simulink model "NMPC_6DoF_v1"  (R2022b)
settings: Solver=ode45  StartTime=0.0  StopTime=30  FixedStep=0.01  RelTol=1e-3
undefined symbols (not defined in the file): beta, e0_0, e1_0, e2_0, e3_0, eul0, G0, gamma, gc, geometry, Js, Js0, K_lqrq, m_dry, m_fuel, m_full, m_max, mass, omega0, pos0, r_cg, rcgs, ref_eul, Tensors, vel0
libraries: sharedtransform x27, simulink_extras x21, matrix_library x12, sharedutil x2, sharedTrackingLibrary x1, mpclib x1
(part 2 of 2)

== system NMPC_6DoF_v1/6DOF HopperDynamic/Rocket Dynamics 6DOF2/Calculate omega_dot ==
  p q r : Inport
  "I, I_dot" : Inport  Port=2
  Moments : Inport  Port=3
  3x3 Cross Product : sharedutil/3x3 Cross Product  aMode=aMode
  I x w : Subsystem
  I x w1 : Subsystem
  Product2 : Product  Inputs=*/  Multiplication=Matrix(*)  SaturateOnIntegerOverflow=on  OutDataTypeStr=Inherit: Same as first input
  Reshape : Reshape
  Reshape1 : Reshape  OutputDimensionality=Row vector (2-D)
  Selector : Selector  NumberOfDimensions=2  InputPortWidth=2  IndexOptions=Index vector (dialog),Select all  Indices=1:3,-1  OutputSizes=1
  Selector1 : Selector  NumberOfDimensions=2  InputPortWidth=2  IndexOptions=Index vector (dialog),Select all  Indices=4:6,-1  OutputSizes=1
  Selector2 : Selector  NumberOfDimensions=2  InputPortWidth=2  IndexOptions=Index vector (dialog),Select all  Indices=1:3,-1  OutputSizes=1
  Sum2 : Sum  Inputs=+--  SaturateOnIntegerOverflow=on
  pdot qdot rdot : Outport  VectorParamsAs1DForOutWhenUnconnected=off
  wires:
  "I, I_dot"/1 -> Selector1/1, Selector2/1, Selector/1
  Selector/1 -> I x w/2(Inertia)
  I x w/1(I * w) -> 3x3 Cross Product/2
  p q r/1 -> I x w1/2(p q r), 3x3 Cross Product/1, I x w/1(p q r)
  Moments/1 -> Sum2/1
  I x w1/1(Id * w) -> Sum2/2
  3x3 Cross Product/1 -> Sum2/3
  Sum2/1 -> Reshape1/1
  Reshape/1 -> pdot qdot rdot/1
  Selector2/1 -> Product2/2
  Reshape1/1 -> Product2/1
  Product2/1 -> Reshape/1
  Selector1/1 -> I x w1/1(I_dot)

== system NMPC_6DoF_v1/6DOF HopperDynamic/Rocket Dynamics 6DOF2/Determine Force, Mass & Inertia ==
  forces : Inport
  "mass " : Inport  Port=2
  I : Inport  Port=3
  I_dot : Inport  Port=4
  Matrix Concatenation : Concatenate  Mode=Multidimensional array
  "forces " : Outport  PortDimensions=3  VectorParamsAs1DForOutWhenUnconnected=off
  mass : Outport  Port=2  VectorParamsAs1DForOutWhenUnconnected=off
  "I, I_dot " : Outport  Port=3  VectorParamsAs1DForOutWhenUnconnected=off
  wires:
  "mass "/1 -> mass/1
  I/1 -> Matrix Concatenation/1
  I_dot/1 -> Matrix Concatenation/2
  Matrix Concatenation/1 -> "I, I_dot "/1
  forces/1 -> "forces "/1

== system NMPC_6DoF_v1/6DOF HopperDynamic/Rocket Dynamics 6DOF2/transform to Inertial axes ==
  x y z : Inport
  transform coefficients : Inport  Port=2
  Product : Product  Multiplication=Matrix(*)  InputSameDT=on  SaturateOnIntegerOverflow=on  OutDataTypeStr=Inherit: Same as first input
  Reshape1 : Reshape  OutputDimensionality=Column vector (2-D)
  Reshape2 : Reshape
  Ve : Outport  VectorParamsAs1DForOutWhenUnconnected=off
  wires:
  transform coefficients/1 -> Product/1
  Product/1 -> Reshape2/1
  Reshape1/1 -> Product/2
  x y z/1 -> Reshape1/1
  Reshape2/1 -> Ve/1

== system NMPC_6DoF_v1/6DOF HopperDynamic/Rocket Dynamics 6DOF2/Calculate DCM & Euler Angles/phi_dot theta_dot psi_dot ==
  p q r : Inport
  phi theta psi : Inport  Port=2
  Mux1 : Mux  Inputs=[3 3 3]
  Mux2 : Mux  Inputs=3
  phi psi theta : Selector  InputPortWidth=3  IndexOptions=Index vector (dialog)  Indices=[1 3 2]  OutputSizes=1
  phidot : Fcn  Expr=u[1]+(u[2]*u[4]+u[3]*u[7])*(u[5]/u[8])
  psidot : Fcn  Expr=u[2]*u[7]-u[3]*u[4]
  sincos : Trigonometry  Operator=sincos
  thetadot : Fcn  Expr=(u[2]*u[4]+u[3]*u[7])/u[8]
  phidot thetadot psidot : Outport
  wires:
  phidot/1 -> Mux2/1
  thetadot/1 -> Mux2/2
  sincos/1 -> Mux1/2
  Mux1/1 -> psidot/1, thetadot/1, phidot/1
  p q r/1 -> Mux1/1
  sincos/2 -> Mux1/3
  psidot/1 -> Mux2/3
  phi theta psi/1 -> phi psi theta/1
  phi psi theta/1 -> sincos/1
  Mux2/1 -> phidot thetadot psidot/1

== system NMPC_6DoF_v1/6DOF HopperDynamic/Rocket Dynamics 6DOF2/Calculate DCM & Euler Angles/qdot ==
  p q r : Inport
  q0 q1 q2 q3 : Inport  Port=2
  Constant : Constant
  Dot Product : DotProduct  InputSameDT=off  OutDataTypeStr=Inherit: Inherit via internal rule
  High Gain Quaternion Normalization : Gain  Gain=k_quat  SaturateOnIntegerOverflow=on  OutDataTypeStr=Inherit: Same as input  ParamDataTypeStr=Inherit: Same as input
  Mux1 : Mux  Inputs=[3 4 1]
  Mux2 : Mux
  Sum : Sum  Inputs=|+-  InputSameDT=on  SaturateOnIntegerOverflow=on  OutDataTypeStr=Inherit: Same as first input
  q0dot : Fcn  Expr=-0.5 * ( u[5]*u[1]+u[6]*u[2]+u[7]*u[3] ) + u[8]*u[4]
  q1dot : Fcn  Expr=0.5 * ( u[4]*u[1]+u[6]*u[3]-u[7]*u[2] ) + u[8]*u[5]
  q2dot : Fcn  Expr=0.5 * ( u[4]*u[2]+u[7]*u[1]-u[5]*u[3] ) + u[8]*u[6]
  q3dot : Fcn  Expr=0.5 * ( u[4]*u[3]+u[5]*u[2]-u[6]*u[1] ) + u[8]*u[7]
  qdot : Outport  InitialOutput=0  VectorParamsAs1DForOutWhenUnconnected=off
  wires:
  q0dot/1 -> Mux2/1
  Sum/1 -> High Gain Quaternion Normalization/1
  Constant/1 -> Sum/1
  p q r/1 -> Mux1/1
  High Gain Quaternion Normalization/1 -> Mux1/3
  Dot Product/1 -> Sum/2
  q0 q1 q2 q3/1 -> Dot Product/1, Dot Product/2, Mux1/2
  Mux2/1 -> qdot/1
  q3dot/1 -> Mux2/4
  Mux1/1 -> q2dot/1, q3dot/1, q0dot/1, q1dot/1
  q2dot/1 -> Mux2/3
  q1dot/1 -> Mux2/2

== system NMPC_6DoF_v1/6DOF HopperDynamic/Rocket Dynamics 6DOF2/Calculate omega_dot/I x w ==
  p q r : Inport
  Inertia : Inport  Port=2
  Product : Product  Multiplication=Matrix(*)  InputSameDT=on  SaturateOnIntegerOverflow=on  OutDataTypeStr=Inherit: Same as first input
  Reshape1 : Reshape  OutputDimensionality=Column vector (2-D)
  Reshape2 : Reshape
  I * w : Outport  VectorParamsAs1DForOutWhenUnconnected=off
  wires:
  Inertia/1 -> Product/1
  Reshape1/1 -> Product/2
  Product/1 -> Reshape2/1
  p q r/1 -> Reshape1/1
  Reshape2/1 -> I * w/1

== system NMPC_6DoF_v1/6DOF HopperDynamic/Rocket Dynamics 6DOF2/Calculate omega_dot/I x w1 ==
  I_dot : Inport
  p q r : Inport  Port=2
  Product : Product  Multiplication=Matrix(*)  InputSameDT=on  SaturateOnIntegerOverflow=on  OutDataTypeStr=Inherit: Same as first input
  Reshape1 : Reshape  OutputDimensionality=Column vector (2-D)
  Reshape2 : Reshape
  Id * w : Outport  VectorParamsAs1DForOutWhenUnconnected=off
  wires:
  I_dot/1 -> Product/1
  Reshape1/1 -> Product/2
  Product/1 -> Reshape2/1
  p q r/1 -> Reshape1/1
  Reshape2/1 -> Id * w/1

== matlab function NMPC_6DoF_v1/6DOF HopperDynamic/MATLAB Function ==
  data: m_current input; J output; mass input; Tensors input
function J = Tensor_of_Inertia(m_current, mass, Tensors)
    % interpolation components of tensor of inertia
    J = tensor_interpolation(m_current, mass, Tensors);
end

== matlab function NMPC_6DoF_v1/Actuator Forces/Center of Mass1 ==
  data: m_input input; CoM output; mass input; rcgs input
function CoM = current_CoM(m_input, mass, rcgs)
    CoM = mass_center_interpolate(m_input, mass, rcgs);
